simulink model "minMaxNeuralProcessorSplit"  (R2012b)
settings: Solver=FixedStepDiscrete  StartTime=0.0  StopTime=10.0  FixedStep=0.001  RelTol=1e-3
settings Model: BufferReuse=off  Creator=gilja  LastModifiedBy=NPTL
settings SolverCC: EnableConcurrentExecution=on  ConcurrentTasks=on
settings DataIOCC: SaveOutput=off  SignalLogging=off  DSMLogging=off  SaveTime=off
settings OptimizationCC: InlineParams=on  InlineInvariantSignals=on  OptimizeBlockIOStorage=off  BufferReuse=off  ExpressionFolding=off  LocalBlockOutputs=off
settings HardwareCC: ProdIntDivRoundTo=Zero  ProdEndianess=LittleEndian  ProdHWDeviceType=Generic->32-bit x86 compatible
settings ModelReferenceCC: ModelReferenceMinAlgLoopOccurrences=on
settings RTWCC: SystemTargetFile=xpctarget.tlc  TemplateMakefile=xpc_default_tmf  Description=xPC Target  ProcessScript=xpctarget_make_rtw_hook  RTWCompilerOptimization=On
settings CodeAppCC: MaxIdLength=62
settings xpcTargetCC: TargetFcnLib=ansi_tfl_table_tmw.mat  CodeReplacementLibrary=XPC_BLAS  ParMdlRefBuildCompliant=on  ConcurrentExecutionCompliant=on  CombineSignalStateStructs=off  GRTInterface=on  xPCTaskExecutionProfile=on  xPCRL32EventNumber=5000  xPCisDownloadable=off  xPCLoadParamSetFile=off  xPCConcurrentTasks=off  xPCEnableSFAnimation=off

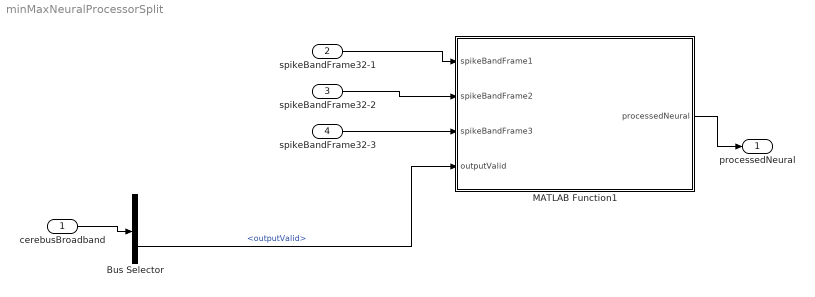
== system minMaxNeuralProcessorSplit ==
  cerebusBroadband : Inport  OutDataTypeStr=Bus: cerebusBroadband
  spikeBandFrame32-1 : Inport  Port=2  OutDataTypeStr=single  PortDimensions=[30 32]
  spikeBandFrame32-2 : Inport  Port=3  OutDataTypeStr=single  PortDimensions=[30 32]
  spikeBandFrame32-3 : Inport  Port=4  OutDataTypeStr=single  PortDimensions=[30 32]
  Bus Selector : BusSelector  OutputSignals=cerebusFrame,outputValid
  MATLAB Function1 : MATLAB Function  TreatAsAtomicUnit=on
  processedNeural : Outport  OutDataTypeStr=Bus: processedNeural  BusOutputAsStruct=on
  wires:
  MATLAB Function1/1(processedNeural) -> processedNeural/1
  cerebusBroadband/1 -> Bus Selector/1
  Bus Selector/2 -> MATLAB Function1/4(outputValid)  "<outputValid>"
  spikeBandFrame32-1/1 -> MATLAB Function1/1(spikeBandFrame1)
  spikeBandFrame32-2/1 -> MATLAB Function1/2(spikeBandFrame2)
  spikeBandFrame32-3/1 -> MATLAB Function1/3(spikeBandFrame3)

== matlab function minMaxNeuralProcessorSplit/MATLAB Function1 ==
  data: spikeBandFrame1 input; spikeBandFrame2 input; spikeBandFrame3 input; outputValid input; xpcConstants parameter; processedNeural output Bus: processedNeural
function processedNeural = extractNerualMaxMin(spikeBandFrame1, spikeBandFrame2, spikeBandFrame3, outputValid, xpcConstants)
%#codegen
persistent bufferMeanSquared bufferIdx bufferCnt bufferReady;
persistent spikeBandFrame;

if(isempty(bufferCnt))
    bufferCnt = 0;
    bufferIdx = 0;
    spikeBandFrame = single(zeros(size(spikeBandFrame1,1), size(spikeBandFrame1,2)*3));
    bufferMeanSquared = single(zeros(2, size(spikeBandFrame, 2)));
    bufferReady = false;
end

spikeBandFrame = horzcat(single(spikeBandFrame1),single(spikeBandFrame2),single(spikeBandFrame3));

if (bufferCnt == xpcConstants.RMSperiod)
    bufferIdx = 1 - bufferIdx;
    bufferMeanSquared(2-bufferIdx, :) = 0;
    bufferCnt = 0;
    bufferReady = true;
end


bufferMeanSquared(2-bufferIdx, :) = bufferMeanSquared(2-bufferIdx, :) + mean(spikeBandFrame.^2) / xpcConstants.RMSperiod; 
bufferCnt = bufferCnt + 1;

if(bufferReady && (bufferCnt <= size(spikeBandFrame, 2)))
    processedNeural.meanSquared = bufferMeanSquared(bufferIdx + 1, bufferCnt);
    processedNeural.meanSquaredChannel = uint8(bufferCnt);
else
    processedNeural.meanSquared = single(0);
    processedNeural.meanSquaredChannel = uint8(0);
end
   
   
[processedNeural.minSpikeBand tmpMin] = min(spikeBandFrame);
processedNeural.minSpikeBandInd = uint8(tmpMin);
[processedNeural.maxSpikeBand tmpMax] = max(spikeBandFrame);
processedNeural.maxSpikeBandInd = uint8(tmpMax);
processedNeural.outputValid = outputValid;
